simulink model "MCASSimulation__exp"  (R2022b)
settings: Solver=VariableStepAuto  StartTime=0.0  StopTime=350  RelTol=1e-3
model workspace (MAT data in the model file):
  ASd = 1
values from neighbouring files (symbols this model uses):
  sortedParams = table2struct(sortedT)    [RunSimulations.m]    (also in no_anomolies_run_handler.m)
libraries: slpidlib x12, simulink_extras x3
(part 2 of 4)

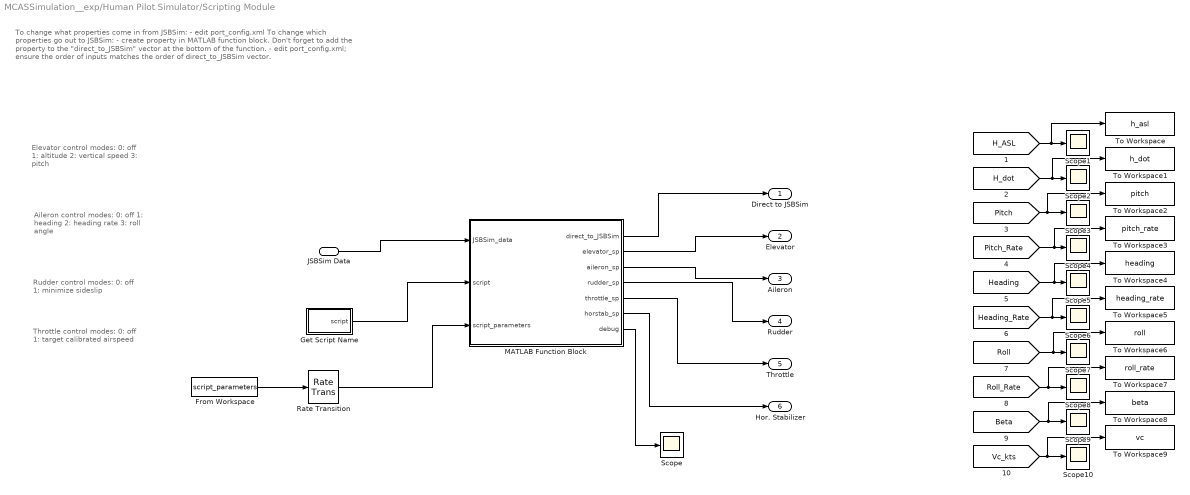
== system MCASSimulation__exp/Human Pilot Simulator/Scripting Module ==
  note: To change what properties come in from JSBSim:
      | - edit port_config.xml
      |
      | To change which properties go out to JSBSim:
      | - create property in MATLAB function block. Don't forget to add the property to the "direct_to_JSBSim" vector at the bottom of the function.
      | - edit port_config.xml; ensure the order of inputs matches the order of direct_to_JSBSim vector.
  note: Throttle control modes:
      | 0: off
      | 1: target calibrated airspeed
  note: Rudder control modes:
      | 0: off
      | 1: minimize sideslip
  note: Elevator control modes:
      | 0: off
      | 1: altitude
      | 2: vertical speed
      | 3: pitch
  note: Aileron control modes:
      | 0: off
      | 1: heading
      | 2: heading rate
      | 3: roll angle
  JSBSim Data : Inport
  From Workspace : FromWorkspace  VariableName=script_parameters
  Get Script Name : Subsystem
  MATLAB Function Block : MATLAB Function  TreatAsAtomicUnit=on
  Rate Transition : RateTransition  OutPortSampleTime=8.3333e-03
  Scope{,1..10} (11 alike) : Scope
  To Workspace : ToWorkspace  VariableName=h_asl  SaveFormat=Timeseries  SampleTime=-1
  To Workspace1 : ToWorkspace  VariableName=h_dot  SaveFormat=Timeseries  SampleTime=-1
  To Workspace2 : ToWorkspace  VariableName=pitch  SaveFormat=Timeseries  SampleTime=-1
  To Workspace3 : ToWorkspace  VariableName=pitch_rate  SaveFormat=Timeseries  SampleTime=-1
  To Workspace4 : ToWorkspace  VariableName=heading  SaveFormat=Timeseries  SampleTime=-1
  To Workspace5 : ToWorkspace  VariableName=heading_rate  SaveFormat=Timeseries  SampleTime=-1
  To Workspace6 : ToWorkspace  VariableName=roll  SaveFormat=Timeseries  SampleTime=-1
  To Workspace7 : ToWorkspace  VariableName=roll_rate  SaveFormat=Timeseries  SampleTime=-1
  To Workspace8 : ToWorkspace  VariableName=beta  SaveFormat=Timeseries  SampleTime=-1
  To Workspace9 : ToWorkspace  VariableName=vc  SaveFormat=Timeseries  SampleTime=-1
  Direct to JSBSim : Outport
  Elevator : Outport  Port=2
  Aileron : Outport  Port=3
  Rudder : Outport  Port=4
  Throttle : Outport  Port=5
  Hor. Stabilizer : Outport  Port=6
  wires:
  MATLAB Function Block/5(throttle_sp) -> Throttle/1
  MATLAB Function Block/3(aileron_sp) -> Aileron/1
  MATLAB Function Block/4(rudder_sp) -> Rudder/1
  MATLAB Function Block/2(elevator_sp) -> Elevator/1
  MATLAB Function Block/1(direct_to_JSBSim) -> Direct to JSBSim/1
  [Roll] -> To Workspace6/1, Scope7/1
  [Roll_Rate] -> To Workspace7/1, Scope8/1
  [Heading_Rate] -> To Workspace5/1, Scope6/1
  [Vc_kts] -> To Workspace9/1, Scope10/1
  [Beta] -> To Workspace8/1, Scope9/1
  [Pitch] -> To Workspace2/1, Scope3/1
  [Pitch_Rate] -> To Workspace3/1, Scope4/1
  [H_ASL] -> To Workspace/1, Scope1/1
  [H_dot] -> To Workspace1/1, Scope2/1
  [Heading] -> To Workspace4/1, Scope5/1
  Get Script Name/1(script) -> MATLAB Function Block/2(script)
  JSBSim Data/1 -> MATLAB Function Block/1(JSBSim_data)
  MATLAB Function Block/6(horstab_sp) -> Hor. Stabilizer/1
  Rate Transition/1 -> MATLAB Function Block/3(script_parameters)
  From Workspace/1 -> Rate Transition/1
  MATLAB Function Block/7(debug) -> Scope/1

== system MCASSimulation__exp/Human Pilot Simulator/Signal Packing ==
  note: Merges elevator, aileron, rudder, and throttle commands, as well as any other relevant signals, into one signal for sendign to JSBSim. Must interface with JSBSim SFunction port configuration.
  From Scripting : Inport
  Elevator Cmd (norm) : Inport  Port=2
  Aileron Cmd (norm) : Inport  Port=3
  Rudder Cmd (norm) : Inport  Port=4
  Throttle Cmds (norm) : Inport  Port=5
  Stab-Target Diff : Inport  Port=6
  Mux : Mux  Inputs=[-1, 1, 1, 1, 2, 3]
  To JSBSim : Outport
  wires:
  Mux/1 -> To JSBSim/1
  Rudder Cmd (norm)/1 -> Mux/4
  Aileron Cmd (norm)/1 -> Mux/3
  Throttle Cmds (norm)/1 -> Mux/5
  Elevator Cmd (norm)/1 -> Mux/2
  From Scripting/1 -> Mux/1
  Stab-Target Diff/1 -> Mux/6

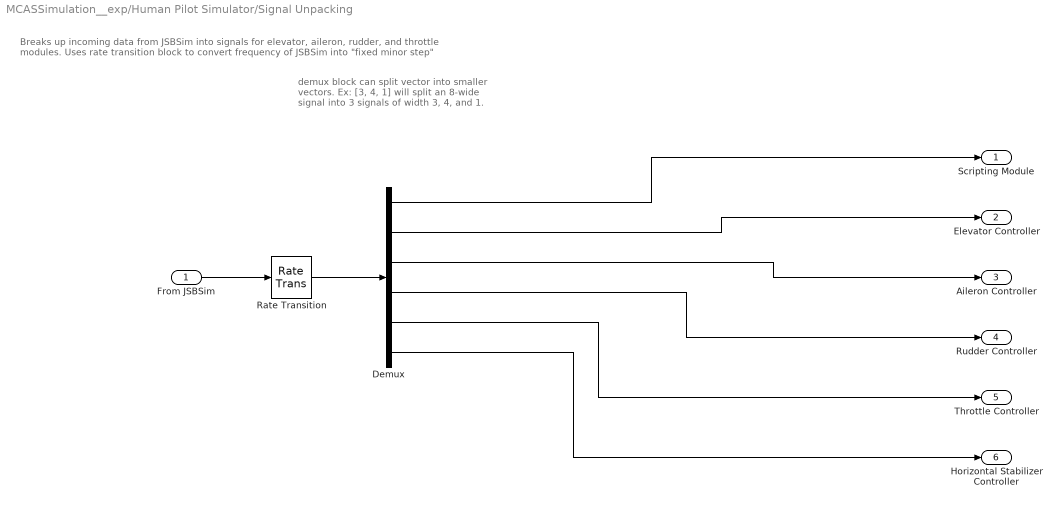
== system MCASSimulation__exp/Human Pilot Simulator/Signal Unpacking ==
  note: demux block can split vector into smaller vectors. Ex: [3, 4, 1] will split an 8-wide signal into 3 signals of width 3, 4, and 1.
  note: Breaks up incoming data from JSBSim into signals for elevator, aileron, rudder, and throttle modules. Uses rate transition block to convert frequency of JSBSim into "fixed minor step"
  From JSBSim : Inport
  Demux : Demux  Outputs=[-1, 5, 4, 1, 1, 1]
  Rate Transition : RateTransition
  Scripting Module : Outport
  Elevator Controller : Outport  Port=2
  Aileron Controller : Outport  Port=3
  Rudder Controller : Outport  Port=4
  Throttle Controller : Outport  Port=5
  Horizontal Stabilizer Controller : Outport  Port=6
  wires:
  From JSBSim/1 -> Rate Transition/1
  Rate Transition/1 -> Demux/1
  Demux/2 -> Elevator Controller/1
  Demux/3 -> Aileron Controller/1
  Demux/4 -> Rudder Controller/1
  Demux/5 -> Throttle Controller/1
  Demux/1 -> Scripting Module/1
  Demux/6 -> Horizontal Stabilizer Controller/1

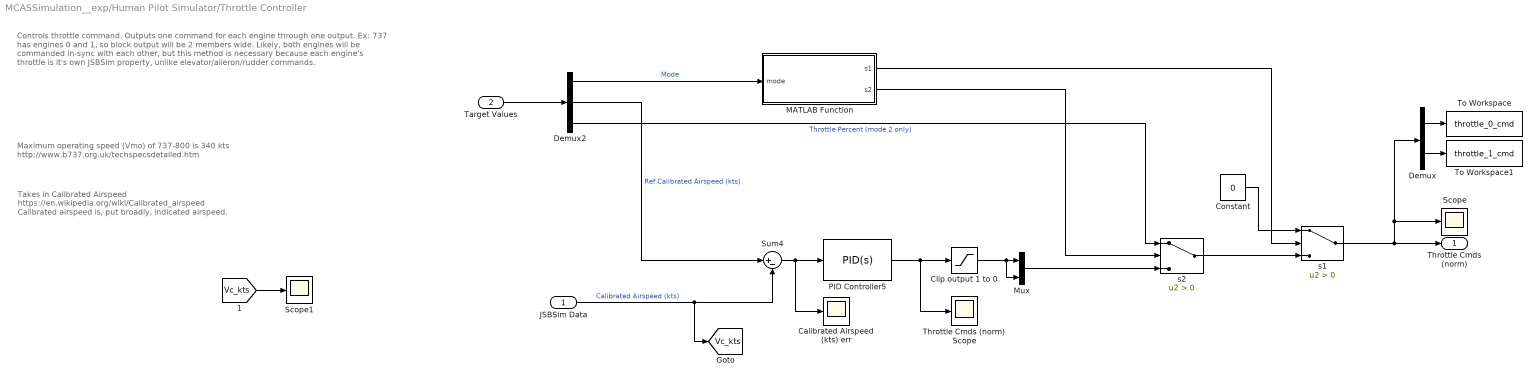
== system MCASSimulation__exp/Human Pilot Simulator/Throttle Controller ==
  note: Maximum operating speed (Vmo) of 737-800 is 340 kts
      | http://www.b737.org.uk/techspecsdetailed.htm
  note: Takes in Calibrated Airspeed
      | https://en.wikipedia.org/wiki/Calibrated_airspeed
      | Calibrated airspeed is, put broadly, indicated airspeed.
  note: Controls throttle command. Outputs one command for each engine through one output.
      |
      | Ex: 737 has engines 0 and 1, so block output will be 2 members wide. Likely, both engines will be commanded in-sync with each other, but this method is necessary because each engine's throttle is it's own JSBSim property, unlike elevator/aileron/rudder commands.
  JSBSim Data : Inport
  Target Values : Inport  Port=2
  Calibrated Airspeed (kts) err : Scope
  Clip output 1 to 0 : Saturate  UpperLimit=1  LowerLimit=0
  Constant : Constant  Value=0
  Demux : Demux  Outputs=2
  Demux2 : Demux  Outputs=3
  MATLAB Function : MATLAB Function  TreatAsAtomicUnit=on
  Mux : Mux  Inputs=2
  PID Controller5 : slpidlib/PID Controller  Controller=PID  Form=Parallel  TimeDomain=Continuous-time  UseExternalTs=off  SampleTime=-1  IntegratorMethod=Forward Euler  FilterMethod=Forward Euler  ControllerParametersSource=internal  P=0.5  I=0.2  UseKiTs=off  D=0.7  N=100  UseFilter=on  TunerSelectOption=Transfer Function Based (PID Tuner App)  InitialConditionSource=internal  InitialConditionForIntegrator=0  InitialConditionForFilter=0  DifferentiatorICPrevScaledInput=0  ExternalReset=none  TrackingMode=off  Kt=1  LimitOutput=on  SatLimitsSource=internal  UpperSaturationLimit=1  LowerSaturationLimit=0  LinearizeAsGain=on  AntiWindupMode=clamping  Kb=1  LimitIntegrator=off  UpperIntegratorSaturationLimit=inf  LowerIntegratorSaturationLimit=-inf  POutMin=[]  POutMax=[]  IOutMin=[]  IOutMax=[]  DOutMin=[]  DOutMax=[]  NOutMin=[]  NOutMax=[]  SumOutMin=[]  SumOutMax=[]  SaturationOutMin=[]  SaturationOutMax=[]  PParamMin=[]  PParamMax=[]  IParamMin=[]  IParamMax=[]  DParamMin=[]  DParamMax=[]  NParamMin=[]  NParamMax=[]  KbParamMin=[]  KbParamMax=[]  KtParamMin=[]  KtParamMax=[]  KbOutMin=[]  KbOutMax=[]  KtOutMin=[]  KtOutMax=[]  IntegratorOutMin=[]  IntegratorOutMax=[]  FilterOutMin=[]  FilterOutMax=[]  SumI1OutMin=[]  SumI1OutMax=[]  SumI2OutMin=[]  SumI2OutMax=[]  SumI3OutMin=[]  SumI3OutMax=[]  SumI4OutMin=[]  SumI4OutMax=[]  SumDOutMin=[]  SumDOutMax=[]  DifferentiatorOutMin=[]  DifferentiatorOutMax=[]  FilterDiffOutCoefMin=[]  FilterDiffOutCoefMax=[]  ReciprocalOutMin=[]  ReciprocalOutMax=[]  SumDenOutMin=[]  SumDenOutMax=[]  SumNumOutMin=[]  SumNumOutMax=[]  DivideOutMin=[]  DivideOutMax=[]  UdiffTsProdOutMin=[]  UdiffTsProdOutMax=[]  NTsProdOutMin=[]  NTsProdOutMax=[]  UintegralTsProdOutMin=[]  UintegralTsProdOutMax=[]  UngainTsProdOutMin=[]  UngainTsProdOutMax=[]  ClampingZeroOutDataTypeStr=Inherit: Inherit via back propagation  ClampingZeroOutMin=[]  ClampingZeroOutMax=[]  FilterDenConstantOutDataTypeStr=Inherit: Inherit via back propagation  FilterDenConstantOutMin=[]  FilterDenConstantOutMax=[]  PCopyOutDataTypeStr=Inherit: Inherit via back propagation  PCopyOutMin=[]  PCopyOutMax=[]  NCopyOutDataTypeStr=Inherit: Inherit via back propagation  NCopyOutMin=[]  NCopyOutMax=[]  IntegratorContinuousStateAttributes=''  IntegratorStateMustResolveToSignalObject=off  IntegratorRTWStateStorageClass=Auto  FilterContinuousStateAttributes=''  FilterStateMustResolveToSignalObject=off  FilterRTWStateStorageClass=Auto  ParallelPVariant=InternalParameters  IdealPVariant=Disabled  IVariant=InternalParameters  DVariant=InternalParameters  IntegratorVariant=Continuous  SatVariant=Enabled  AWVariant=ContClampingParallel  PCopyVariant=Disabled  TRVariant=Disabled  FdbkBlocksVariant=Forward  IdealPFdbkVariant=Disabled  SatFdbkVariant=Disabled  DerivativeFilterVariant=ContFilter  NVariant=InternalParameters  NCopyVariant=Disabled  FilterICVariant=InternalICsFilter  IntegratorICVariant=InternalICs  ExternalResetVariant=Disabled  TRSumVariant=Passthrough  SumFdbkVariant=Disabled  SumVariant=Sum_PID  TsampFilterVariant=InternalTs  TsampNgainVariant=Passthrough  TsampIntegralVariant=Passthrough  ExternalSaturationOutDataTypeStr=Inherit: Same as second input
  Scope : Scope
  Scope1 : Scope
  Sum4 : Sum  Inputs=|+-
  Throttle Cmds (norm) Scope : Scope
  To Workspace : ToWorkspace  VariableName=throttle_0_cmd  SaveFormat=Timeseries  SampleTime=-1
  To Workspace1 : ToWorkspace  VariableName=throttle_1_cmd  SaveFormat=Timeseries  SampleTime=-1
  s1 : Switch  Criteria=u2 > Threshold  SaturateOnIntegerOverflow=off  InputSameDT=off
  s2 : Switch  Criteria=u2 > Threshold  SaturateOnIntegerOverflow=off  InputSameDT=off
  Throttle Cmds (norm) : Outport
  tag scope: Vc_kts=global
  wires:
  Clip output 1 to 0/1 -> Mux/2, Mux/1
  JSBSim Data/1 -> [Vc_kts], Sum4/2  "Calibrated Airspeed (kts)"
  Sum4/1 -> Calibrated Airspeed (kts) err/1, PID Controller5/1
  PID Controller5/1 -> Clip output 1 to 0/1, Throttle Cmds (norm) Scope/1
  Mux/1 -> s2/3
  s1/1 -> Demux/1, Scope/1, Throttle Cmds (norm)/1
  MATLAB Function/1(s1) -> s1/2
  Demux2/2 -> Sum4/1  "Ref Calibrated Airspeed (kts)"
  Demux2/1 -> MATLAB Function/1(mode)  "Mode"
  Target Values/1 -> Demux2/1
  [Vc_kts] -> Scope1/1
  Demux/1 -> To Workspace/1
  Demux/2 -> To Workspace1/1
  Demux2/3 -> s2/1  "Throttle Percent (mode 2 only)"
  s2/1 -> s1/3
  MATLAB Function/2(s2) -> s2/2
  Constant/1 -> s1/1

== system MCASSimulation__exp/MCAS/Get MCAS Name ==
  note: From workspace block likes taking arrays of doubles but not strings. This subsystem takes an array of ASCII doubles from the workspace and converts it to a string.
      |
      | As cumbersome a solution as it seems, it works and is the best solution I can find.
  ASCII to String : ASCIIToString
  Data Type Conversion : DataTypeConversion  OutDataTypeStr=uint8  SaturateOnIntegerOverflow=off  RndMeth=Floor
  From Workspace : FromWorkspace  VariableName=function_block_MCAS
  MCAS : Outport
  wires:
  From Workspace/1 -> Data Type Conversion/1
  Data Type Conversion/1 -> ASCII to String/1
  ASCII to String/1 -> MCAS/1

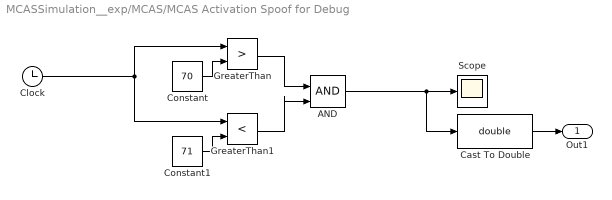
== system MCASSimulation__exp/MCAS/MCAS Activation Spoof for Debug ==
  AND : Logic  IconShape=distinctive  AllPortsSameDT=off  OutDataTypeStr=boolean
  Cast To Double : DataTypeConversion  OutDataTypeStr=double  SaturateOnIntegerOverflow=off  RndMeth=Floor
  Clock : Clock
  Constant : Constant  Value=70
  Constant1 : Constant  Value=71
  GreaterThan : RelationalOperator  Operator=>  OutDataTypeStr=boolean  RndMeth=Simplest  InputSameDT=off
  GreaterThan1 : RelationalOperator  Operator=<  OutDataTypeStr=boolean  RndMeth=Simplest  InputSameDT=off
  Scope : Scope
  Out1 : Outport
  wires:
  Constant1/1 -> GreaterThan1/2
  Clock/1 -> GreaterThan/1, GreaterThan1/1
  Constant/1 -> GreaterThan/2
  GreaterThan/1 -> AND/1
  GreaterThan1/1 -> AND/2
  AND/1 -> Scope/1, Cast To Double/1
  Cast To Double/1 -> Out1/1

== system MCASSimulation__exp/Human Pilot Simulator/Aileron Controller/Turn Direction Correction ==
  note: If heading error > 180
      | 	subtract 360
      | If heading error < -180
      | 	Add 360
      |
      | This is to prevent the plane from taking the 'long way around' when making a turn (i.e. a 270 degree left turn instead of a 90 degree right turn)
  In1 : Inport
  If : If  IfExpression=u1 > 180  ElseIfExpressions=u1 < -180
  If Action Subsystem : Subsystem  TreatAsAtomicUnit=on
  If Action Subsystem1 : Subsystem  TreatAsAtomicUnit=on
  If Action Subsystem2 : Subsystem  TreatAsAtomicUnit=on
  Merge : Merge  Inputs=3
  Scope : Scope
  Scope1 : Scope
  Out1 : Outport
  wires:
  In1/1 -> If/1, Scope/1, If Action Subsystem1/1(In1), If Action Subsystem/1(In1), If Action Subsystem2/1(In1)  "Heading Err (deg)"
  If/3 -> If Action Subsystem/Action
  If Action Subsystem/1(Out1) -> Merge/3
  If/2 -> If Action Subsystem1/Action
  Merge/1 -> Scope1/1, Out1/1
  If Action Subsystem1/1(Out1) -> Merge/2
  If/1 -> If Action Subsystem2/Action
  If Action Subsystem2/1(Out1) -> Merge/1

== system MCASSimulation__exp/Human Pilot Simulator/Scripting Module/Get Script Name ==
  note: From workspace block likes taking arrays of doubles but not strings. This subsystem takes an array of ASCII doubles from the workspace and converts it to a string.
      |
      | As cumbersome a solution as it seems, it works and is the best solution I can find.
  ASCII to String : ASCIIToString
  Data Type Conversion : DataTypeConversion  OutDataTypeStr=uint8  SaturateOnIntegerOverflow=off  RndMeth=Floor
  From Workspace : FromWorkspace  VariableName=function_block_script
  script : Outport
  wires:
  From Workspace/1 -> Data Type Conversion/1
  Data Type Conversion/1 -> ASCII to String/1
  ASCII to String/1 -> script/1

== system MCASSimulation__exp/Human Pilot Simulator/Aileron Controller/Turn Direction Correction/If Action Subsystem ==
  In1 : Inport
  Action Port : ActionPort  ActionPortLabel=else
  Out1 : Outport
  wires:
  In1/1 -> Out1/1

== system MCASSimulation__exp/Human Pilot Simulator/Aileron Controller/Turn Direction Correction/If Action Subsystem1 ==
  In1 : Inport
  Action Port : ActionPort  ActionPortLabel=elseif(u1 < -180)
  Add : Sum
  Constant : Constant  Value=360
  Out1 : Outport
  wires:
  In1/1 -> Add/1
  Constant/1 -> Add/2
  Add/1 -> Out1/1

== system MCASSimulation__exp/Human Pilot Simulator/Aileron Controller/Turn Direction Correction/If Action Subsystem2 ==
  In1 : Inport
  Action Port : ActionPort  ActionPortLabel=if(u1 > 180)
  Constant : Constant  Value=360
  Subtract : Sum  Inputs=+-
  Out1 : Outport
  wires:
  In1/1 -> Subtract/1
  Constant/1 -> Subtract/2
  Subtract/1 -> Out1/1

== matlab function MCASSimulation__exp/MCAS/MCAS Select ==
  data: MCAS input; pilot_control_in input; anomaly_input input; sensor_input input; pilot_control_out output; MCAS_control_out output; MCAS_firing output; MCAS_cooldown output
function [pilot_control_out, MCAS_control_out, MCAS_firing, MCAS_cooldown] = mcas(MCAS, pilot_control_in, anomaly_input, sensor_input)
    % Default for when MCAS does not activate.
    pilot_control_out = pilot_control_in;
    MCAS_control_out = realmin;
    MCAS_firing = 0;

    time_sec = sensor_input(1);

    flaps = anomaly_input(1);
    AoA_r = anomaly_input(2);
    AoA_l = anomaly_input(3);
    h_dot = anomaly_input(4);
    theta = anomaly_input(5);
    MCAS_is_active = sensor_input(14);
    MCAS_cooldown = sensor_input(15);

    % nonnormal means that the flight deviates from checklists.
    persistent nonnormal;
    persistent nonactivate;
    persistent has_triggered;

    if isempty(nonnormal)
        nonnormal = false;
        nonactivate = true;
        has_triggered = false;
    end

    if time_sec <= 30
        return;
    end
       
    switch MCAS

        case "none"
            return;

        case "mcas_old"
            % Assess if MCAS should be activated.
            if AoA_r >= 17
                MCAS_firing = 1;
            end
            return;

        case "mcas_old_adaptive"
            % Assess if MCAS should be activated.
            if AoA_r >= 17
                MCAS_firing = 1;
            end

            if nonactivate && MCAS_firing == 1 && MCAS_is_active == 1
                % Activate MCAS normally.
                nonactivate = false;
                has_triggered = true;
            elseif ~nonactivate && has_triggered && MCAS_firing == 1 && MCAS_is_active == 0
                has_triggered = false;
            elseif ~nonactivate && ~has_triggered && MCAS_firing == 1 && MCAS_is_active == 1
                % Increase cooldown.
                MCAS_cooldown = MCAS_cooldown + 5;
                has_triggered = true;
            elseif ~nonactivate && MCAS_firing ~= 1 && MCAS_is_active ~= 1
                % Signal to reset cooldown and remove activation.
                MCAS_cooldown = 0;
                nonactivate = true;
                has_triggered = false;
            end

            return;

        % Documentation for how the new MCAS works:
        % https://www.boeing.com/commercial/737max/737-max-software-updates.page
        case "mcas_new"

            % Assess if MCAS should be activated.
            if AoA_r >= 17 || AoA_l >= 17

                % Flaps retracted and AoA disagree
                if flaps < 2 && abs(AoA_r - AoA_l) >= 5.5
                    % Do not activate MCAS.
                    return;
                end

                if nonnormal && nonactivate
                    % Activate MCAS once.
                    nonactivate = false;
                    MCAS_firing = 1;
                    return;
                elseif nonnormal && ~nonactivate
                    % Do not activate MCAS
                    return;
                elseif ~nonnormal && ~nonactivate
                    % Reenage to be activated.
                    nonactivate = true;
                end

                if abs(pilot_control_out(7)) > 0.1
                    pilot_control_out(13) = 1;
                end

                % Normal MCAS operation.
                % TODO: Do not allow to be more than max elevator control.
                MCAS_firing = 1;
                return;
            end
            return;
        
        % https://rgl.faa.gov/Regulatory_and_Guidance_Library/rgad.nsf/AOCADSearch/FB91ABC41EF06432862586260051E5DF?OpenDocument
        case "faa_mcas"
            return;
    
        case "sa_mcas_regression"
            % Assess if MCAS should be activated.
            if AoA_r >= 17 || AoA_l >= 17

                est_theta = h_dot*0.1242454 + 4.41805269640706;
                est_AoA = theta*0.01582719 + 4.37842859503393;

                
                if abs(AoA_r - AoA_l) >= 5.5
                    if abs(est_theta - theta) <= 0.20471732629225162*2
                        if abs(est_AoA - AoA_r) <= 0.18450947032615*2 && AoA_r >= 17
                            MCAS_firing = 1;
                        elseif abs(est_AoA - AoA_l) <= 0.18450947032615*2 && AoA_l >= 17
                            MCAS_firing = 1;
                        end
                    end
                else
                    MCAS_firing = 1;
                end
            end

            return;

        %%%
        % alphax = tan^-1(w/U) = w/U0
        % alpha = 
        %
        %
        case "sa_mcas"

            %alpha_mf = atan(u/v);
%             alpha_m = 

            % Assess if MCAS should be activated.
            if AoA_r >= 17 || AoA_l >= 17

                est_theta = h_dot*0.1242454 + 4.41805269640706;
                est_AoA = theta*0.01582719 + 4.37842859503393;

                
                if abs(AoA_r - AoA_l) >= 5.5
                    if abs(est_theta - theta) <= 0.20471732629225162*2
                        if abs(est_AoA - AoA_r) <= 0.18450947032615*2 && AoA_r >= 17
                            MCAS_firing = 1;
                        elseif abs(est_AoA - AoA_l) <= 0.18450947032615*2 && AoA_l >= 17
                            MCAS_firing = 1;
                        end
                    end
                else
                    MCAS_firing = 1;
                end
            end

            return;

        case "sa_mcas_adaptive_regression"
            % Assess if MCAS should be activated.
            if AoA_r >= 17 || AoA_l >= 17

                est_theta = h_dot*0.1242454 + 4.41805269640706;
                est_AoA = theta*0.01582719 + 4.37842859503393;

                
                if abs(AoA_r - AoA_l) >= 5.5
                    if abs(est_theta - theta) <= 0.20471732629225162*2
                        if abs(est_AoA - AoA_r) <= 0.18450947032615*2 && AoA_r >= 17
                            MCAS_firing = 1;
                        elseif abs(est_AoA - AoA_l) <= 0.18450947032615*2 && AoA_l >= 17
                            MCAS_firing = 1;
                        end
                    end
                else
                    MCAS_firing = 1;
                end
            end

            if nonactivate && MCAS_firing == 1 && MCAS_is_active == 1
                % Activate MCAS normally.
                nonactivate = false;
                has_triggered = true;
            elseif ~nonactivate && has_triggered && MCAS_firing == 1 && MCAS_is_active == 0
                has_triggered = false;
            elseif ~nonactivate && ~has_triggered && MCAS_firing == 1 && MCAS_is_active == 1
                % Increase cooldown.
                MCAS_cooldown = MCAS_cooldown + 5;
                has_triggered = true;
            elseif ~nonactivate && MCAS_firing ~= 1 && MCAS_is_active ~= 1
                % Signal to reset cooldown and remove activation.
                MCAS_cooldown = 0;
                nonactivate = true;
                has_triggered = false;
            end
            
            return;
        
        otherwise
            error("MCAS Select: No valid MCAS module selected.");
    end

== matlab function MCASSimulation__exp/Human Pilot Simulator/Elevator Controller/MATLAB Function ==
  data: mode input; s1 output; s2 output; s3 output; s4 output; s5 output
% "0" puts a switch in the "down" position.

function [s1, s2, s3, s4, s5] = mode_selector(mode)

switch mode
    case 0  % off
        s1 = 1;
        s2 = 1;
        s3 = 1;
        s4 = 1;
        s5 = 1;
    case 1  % altitude
        s1 = 0;
        s2 = 0;
        s3 = 0;
        s4 = 1;
        s5 = 0;
    case 2  % vertical speed
        s1 = 0;
        s2 = 0;
        s3 = 0;
        s4 = 1;
        s5 = 1;
    case 3  % pitch
        s1 = 0;
        s2 = 0;
        s3 = 1;
        s4 = 1;
        s5 = 1;
    case 4  % airspeed
        s1 = 0;
        s2 = 0;
        s3 = 0;
        s4 = 0;
        s5 = 1;
    case 5 % direct
        s1 = 0;
        s2 = 1;
        s3 = 0;
        s4 = 0;
        s5 = 1;
    otherwise
        error("elevator mode invalid");

end

== matlab function MCASSimulation__exp/Sensor Anomaly Injection/Injection ==
  settings: updateMethod=DISCRETE
  data: inputdata input; outputdata output; time input; parms input; prev input; currStart data_store_memory
function outputdata = fcn(inputdata, time, parms, prev)

% default
outputdata = inputdata;

if parms(1).InjectionType == 0
    return
end

global currStart;
start = currStart;

persistent recovery_start_val;
persistent diff_start_val;
persistent P;

for i = start : length(parms)

    if time < parms(i).StartTime 
        break;
    elseif time > parms(i).EndTime 
        currStart = i + 1;
        continue;
    else
        switch parms(i).InjectionType
            case 1
                suddenInjection = SuddenInjection(parms(i).Val);
                outputdata(parms(i).SensorIndex) = suddenInjection.injection();
            case 2 
                deltaInjection = DeltaInjection(parms(i).Val);
                outputdata(parms(i).SensorIndex) = deltaInjection.injection(inputdata(parms(i).SensorIndex));
            otherwise
                gradualInjection = GradualInjection(parms(i).Type, parms(i).Coef1, parms(i).Coef2, parms(i).Freq, time);
                outputdata(parms(i).SensorIndex) = gradualInjection.injection(prev(parms(i).SensorIndex));
                recovery_time =  0.75 * (parms(i).EndTime - parms(i).StartTime);
                if time > parms(i).StartTime + recovery_time
                    if isempty(recovery_start_val)
                        recovery_start_val = outputdata(parms(i).SensorIndex);
                        diff_start_val = abs(inputdata(parms(i).SensorIndex) - outputdata(parms(i).SensorIndex));
                    end

                    if abs(recovery_start_val - inputdata(parms(i).SensorIndex)) > 0.1*diff_start_val
                        if ~xor(inputdata(parms(i).SensorIndex) > recovery_start_val, ...
                                recovery_start_val > 0)
                            recovery_start_val = recovery_start_val + 0.05;
                            %recovery_start_val = awgn(recovery_start_val, 0.1);
                        else
                            recovery_start_val = recovery_start_val - 0.05;
                            %recovery_start_val = awgn(recovery_start_val, 0.1);
                        end
                        outputdata(parms(i).SensorIndex) = recovery_start_val;
                    else
                        % Q: small value for noise (usually small)
                        Q = 0.1;  
                        R = 0.2;  
                        
                        % the start point of ending injectionT: T_start = 50,the start sqrt for T: P_start = 2 
                        if isempty(P)
                            P = 2;
                        end
                        %_kalman: best estimate ，_pre: predict
                        T_pre = prev(parms(i).SensorIndex); 
                        P_pre = P + Q; 
                        K = P_pre/(P_pre + R); 
                        outputdata(parms(i).SensorIndex) = T_pre + K*(inputdata(parms(i).SensorIndex) - T_pre); 
                        P = P_pre - K*P_pre;
                    end
                end
        end
    end
end
end
